simulink model "Radar_Acc_ExtSen_CS803"  (Simulink 7.0)
settings: Solver=ode45  StartTime=0  StopTime=50  RelTol=1e-3
libraries: Solver_SF x2, simulink_extras x2, simulink x1
settings Model: Creator=dhall  LastModifiedBy=ywata  ExtModeTrigMode=oneshot  ExtModeArmWhenConnect=off
settings DataIOCC: LimitDataPoints=off  SignalLoggingName=sigsOut
settings OptimizationCC: BooleanDataType=off  LocalBlockOutputs=off
settings DebuggingCC: SaveWithParameterizedLinksMsg=none  SignalResolutionControl=TryResolveAllWithWarning  SolverPrmCheckMsg=none  MultiTaskDSMMsg=warning  MultiTaskCondExecSysMsg=none  StrictBusMsg=None
settings HardwareCC: TargetUnknown=on
settings RTWCC: IncludeERTFirstTime=on
settings GRTTargetCC: TargetFcnLib=ansi_tfl_tmw.mat  CompOptLevelCompliant=off

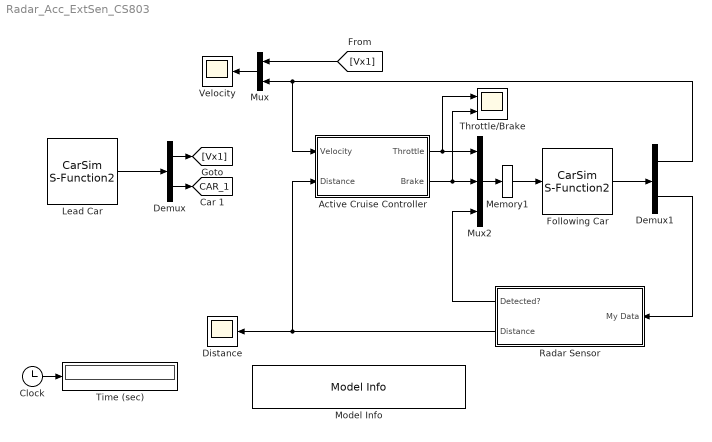
== system Radar_Acc_ExtSen_CS803 ==
  Active Cruise Controller : Subsystem  mask{VX=95, DISTANCE=50}
      mask prompts: VX "Setup Velocity (km/h)"; DISTANCE "Setup Distance (m)"
  Clock : Clock
      settings: Decimation=10
  Demux : Demux  Outputs=[1 3]
  Demux1 : Demux  Outputs=[1 3]
  Distance : Scope
      settings: TickLabels=on  TimeRange=50  YMin=5  YMax=80  DataFormat=Array  SampleTime=100
  Following Car : Solver_SF/CarSim S-Function2  Priority=1  VehicleCode=i_i2  SIMFILE=Radar_Acc_ExtSen_Car_2.sim
      settings: AttributesFormatString=Vehicle Code: %<VehicleCode>
  Lead Car : Solver_SF/CarSim S-Function2  Priority=1  VehicleCode=i_i  SIMFILE=Radar_Acc_ExtSen_Car_1.sim
      settings: AttributesFormatString=Vehicle Code: %<VehicleCode>
  Memory1 : Memory
  Model Info : simulink/Model-Wide Utilities/Model Info  SystemSampleTime=-1  InitialBlockCM=none  BlockCM=none  Frame=on  DisplayStringWithTags=Multi Vehicle Run Adaptive Cruise Control Model  HorizontalTextAlignment=Center  LeftAlignmentValue=0.5  SourceBlockDiagram=tp0f6e990c_25ed_4bdc_ab6a_a57aed6a9554  TagMaxNumber=20
  Mux : Mux  Orientation=left  Inputs=2
  Mux2 : Mux  Inputs=3
  Radar Sensor : Subsystem  Orientation=left  mask{S_ANGLE=10, S_DISTANCE=70}
      mask prompts: S_ANGLE "View Angle (deg)"; S_DISTANCE "Distance Range (m)"
      mask help:
      | An example of a radar sensor. It can detect the distance between the sensor and another object according its position (Xo, Yo).
      |
      | Input parameters are View Angle(deg) and radar detectable distance(m).
      mask init:
      | d_ang= str2double(S_ANGLE)/2;
      | set_param([gcb '/View Angle'], 'Threshold', sprintf('%0.2f', d_ang));
      | set_param([gcb '/L-Radar'], 'Value', S_DISTANCE);
  Throttle/Brake : Scope  NumInputPorts=2
      settings: TickLabels=on  TimeRange=50  YMin=0~0  YMax=1~12.5  DataFormat=Array  MaxDataPoints=50000  SampleTime=100
  Time (sec) : Display
      settings: Format=bank  Decimation=100
  Velocity : Scope
      settings: TickLabels=on  TimeRange=50  YMin=-10  YMax=120  DataFormat=Array  SampleTime=100
  tag scope: CAR_1=global
  wires:
  Clock/1 -> Time (sec)/1
  Active Cruise Controller/2(Brake) -> Mux2/2, Throttle/Brake/2
  Active Cruise Controller/1(Throttle) -> Mux2/1, Throttle/Brake/1
  Demux1/2 -> Radar Sensor/1(My Data)
  Mux/1 -> Velocity/1
  Mux2/1 -> Memory1/1
  Demux/2 -> [CAR_1]
  Demux/1 -> [Vx1]
  Radar Sensor/2(Distance) -> Distance/1, Active Cruise Controller/2(Distance)
  Demux1/1 -> Active Cruise Controller/1(Velocity), Mux/2
  [Vx1] -> Mux/1
  Radar Sensor/1(Detected?) -> Mux2/3
  Lead Car/1 -> Demux/1
  Memory1/1 -> Following Car/1
  Following Car/1 -> Demux1/1

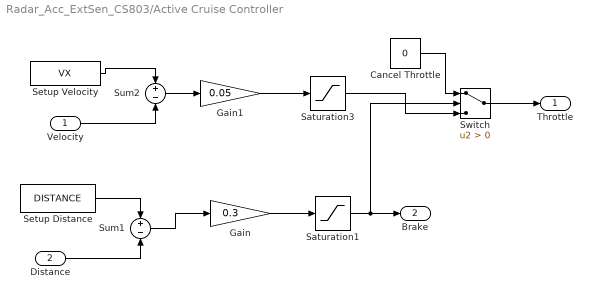
== system Radar_Acc_ExtSen_CS803/Active Cruise Controller ==
  Velocity : Inport  OutDataType=sfix(16)  OutScaling=2^0
  Distance : Inport  Port=2  OutDataType=sfix(16)  OutScaling=2^0
  Cancel Throttle : Constant  Value=0  OutDataType=sfix(16)  OutScaling=2^0
  Gain : Gain  Gain=0.3  ParameterDataType=sfix(16)  ParameterScaling=2^0  OutDataType=sfix(16)  OutScaling=2^0  SaturateOnIntegerOverflow=on
  Gain1 : Gain  Gain=0.05  ParameterDataType=sfix(16)  ParameterScaling=2^0  OutDataType=sfix(16)  OutScaling=2^0  SaturateOnIntegerOverflow=on
  Saturation1 : Saturate  UpperLimit=15  LowerLimit=0
  Saturation3 : Saturate  UpperLimit=1  LowerLimit=0
  Setup Distance : Constant  Value=DISTANCE  OutDataType=sfix(16)  OutScaling=2^0
  Setup Velocity : Constant  Value=VX  OutDataType=sfix(16)  OutScaling=2^0
  Sum1 : Sum  Inputs=+-  OutDataType=sfix(16)  OutScaling=2^0  SaturateOnIntegerOverflow=on  InputSameDT=on
  Sum2 : Sum  Inputs=+-  OutDataType=sfix(16)  OutScaling=2^0  SaturateOnIntegerOverflow=on  InputSameDT=on
  Switch : Switch  Criteria=u2 > Threshold  SaturateOnIntegerOverflow=on
  Throttle : Outport
  Brake : Outport  Port=2
  wires:
  Gain/1 -> Saturation1/1
  Saturation1/1 -> Brake/1, Switch/2
  Setup Velocity/1 -> Sum2/1
  Sum2/1 -> Gain1/1
  Gain1/1 -> Saturation3/1
  Velocity/1 -> Sum2/2
  Switch/1 -> Throttle/1
  Setup Distance/1 -> Sum1/1
  Distance/1 -> Sum1/2
  Sum1/1 -> Gain/1
  Cancel Throttle/1 -> Switch/1
  Saturation3/1 -> Switch/3

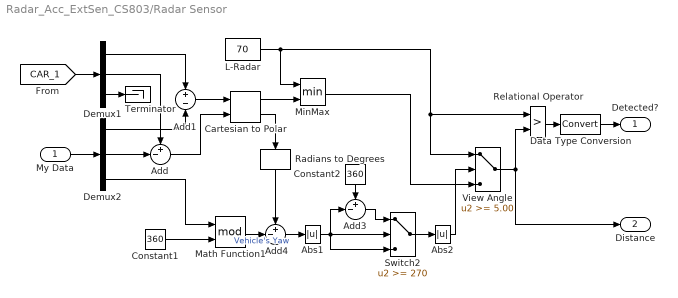
== system Radar_Acc_ExtSen_CS803/Radar Sensor ==
  My Data : Inport  OutDataType=sfix(16)  OutScaling=2^0
  Abs1 : Abs
  Abs2 : Abs
  Add : Sum  Inputs=+-|  OutDataType=sfix(16)  OutScaling=2^-10
  Add1 : Sum  Inputs=+-  OutDataType=sfix(16)  OutScaling=2^-10
  Add3 : Sum  Inputs=+-|  OutDataType=sfix(16)  OutScaling=2^-10
  Add4 : Sum  Inputs=+-|  OutDataType=sfix(16)  OutScaling=2^-10
  Cartesian to Polar : simulink_extras/Transformations/Cartesian to Polar  SystemSampleTime=-1
  Constant1 : Constant  Value=360  OutDataType=sfix(16)  OutScaling=2^0
  Constant2 : Constant  Orientation=down  Value=360  OutDataType=sfix(16)  OutScaling=2^0
  Data Type Conversion : DataTypeConversion  RndMeth=Zero
  Demux1 : Demux  Outputs=3
  Demux2 : Demux  Outputs=3
  L-Radar : Constant  Value=70  OutDataType=sfix(16)  OutScaling=2^0
  Math Function1 : Math  Operator=mod  SaturateOnIntegerOverflow=on
  MinMax : MinMax  Inputs=2  SaturateOnIntegerOverflow=on  InputSameDT=on
  Radians to Degrees : simulink_extras/Transformations/Radians to Degrees  Orientation=down  SystemSampleTime=-1
  Relational Operator : RelationalOperator  Operator=>  LogicOutDataTypeMode=boolean  LogicDataType=double
  Switch2 : Switch  Threshold=270
  Terminator : Terminator
  View Angle : Switch  Threshold=5.00
  Detected? : Outport
  Distance : Outport  Port=2
  wires:
  Demux2/3 -> Math Function1/1
  Constant1/1 -> Math Function1/2
  Add/1 -> Cartesian to Polar/2
  Add1/1 -> Cartesian to Polar/1
  Demux2/1 -> Add1/2
  Demux1/1 -> Add1/1
  Demux2/2 -> Add/2
  Demux1/2 -> Add/1
  Demux1/3 -> Terminator/1
  My Data/1 -> Demux2/1
  [CAR_1] -> Demux1/1
  Math Function1/1 -> Add4/2  "Vehicle's Yaw"
  Add4/1 -> Abs1/1
  Abs1/1 -> Switch2/2, Add3/2, Switch2/3
  Add3/1 -> Switch2/1
  Constant2/1 -> Add3/1
  L-Radar/1 -> MinMax/1, View Angle/1, Relational Operator/1
  MinMax/1 -> View Angle/3
  Switch2/1 -> Abs2/1
  Abs2/1 -> View Angle/2
  View Angle/1 -> Distance/1, Relational Operator/2
  Relational Operator/1 -> Data Type Conversion/1
  Data Type Conversion/1 -> Detected?/1
  Radians to Degrees/1 -> Add4/1
  Cartesian to Polar/1 -> MinMax/2
  Cartesian to Polar/2 -> Radians to Degrees/1
